simulink model "modelP15"  (R2014b)
settings: Solver=ode4  StartTime=0.0  StopTime=TIME_SIM  FixedStep=STEP_SIZE  RelTol=1e-3
values from neighbouring files (symbols this model uses):
  C = [0 0 1]    [mainbis.m]
  K = acker(F,G,Pdisc)    [mainbis.m]
  N = inv(C*inv(eye(3)-Fk)*G)    [mainbis.m]
  Ts = 0.0002    [mainbis.m]
undefined symbols (not defined in the file or in its folder): F, G, Gd
settings Model: Creator=Kate  LastModifiedBy=Kate
settings DataIOCC: SaveState=on

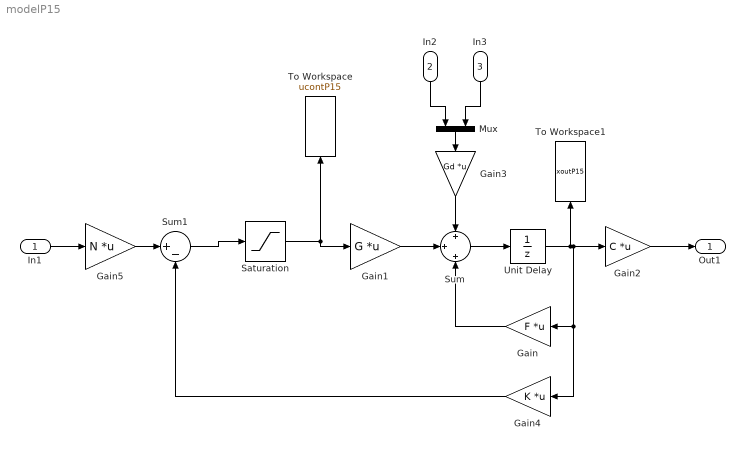
== system modelP15 ==
  In1 : Inport
  In2 : Inport  Port=2
  In3 : Inport  Port=3
  Gain : Gain  Gain=F  Multiplication=Matrix(K*u)
  Gain1 : Gain  Gain=G  Multiplication=Matrix(K*u)
  Gain2 : Gain  Gain=C  Multiplication=Matrix(K*u)
  Gain3 : Gain  Gain=Gd  Multiplication=Matrix(K*u)
  Gain4 : Gain  Gain=K  Multiplication=Matrix(K*u)
  Gain5 : Gain  Gain=N  Multiplication=Matrix(K*u)
  Mux : Mux  Inputs=2
  Saturation : Saturate  UpperLimit=40  LowerLimit=-40
  Sum : Sum  Inputs=+|+|+
  Sum1 : Sum  Inputs=|+-
  To Workspace : ToWorkspace  VariableName=ucontP15  SaveFormat=Timeseries  SampleTime=-1
  To Workspace1 : ToWorkspace  VariableName=xoutP15  SaveFormat=Timeseries  SampleTime=-1
  Unit Delay : UnitDelay  SampleTime=Ts
  Out1 : Outport
  wires:
  Sum/1 -> Unit Delay/1
  Unit Delay/1 -> Gain2/1, Gain4/1, Gain/1, To Workspace1/1
  Gain/1 -> Sum/3
  Gain1/1 -> Sum/2
  Gain2/1 -> Out1/1
  Gain3/1 -> Sum/1
  Mux/1 -> Gain3/1
  In2/1 -> Mux/1
  In3/1 -> Mux/2
  Gain4/1 -> Sum1/2
  In1/1 -> Gain5/1
  Gain5/1 -> Sum1/1
  Sum1/1 -> Saturation/1
  Saturation/1 -> Gain1/1, To Workspace/1
